simulink model "q3_model"  (R2020a)
settings: Solver=VariableStepAuto  StartTime=0.0  StopTime=10.0  RelTol=1e-3
libraries: simulink x1
settings Model: Creator=kiran  LastModifiedBy=kiran

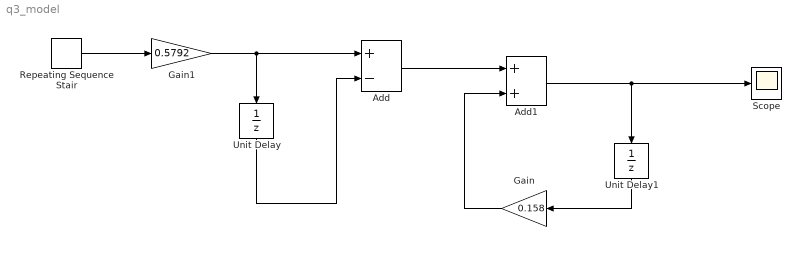
== system q3_model ==
  Add : Sum  Inputs=+-
  Add1 : Sum
  Gain : Gain  Gain=0.158
  Gain1 : Gain  Gain=0.5792
  Repeating Sequence Stair : simulink/Sources/Repeating Sequence Stair  OutValues=[1 0 0 0].'  tsamp=-1  OutMin=[]  OutMax=[]  OutDataTypeStr=double  OutputDataTypeScalingMode=double  OutDataType=fixdt(0,8)  ConRadixGroup=Best Precision: Vector-wise  OutScaling=2^-12
  Scope : Scope
  Unit Delay : UnitDelay  SampleTime=-1  HasFrameUpgradeWarning=on
  Unit Delay1 : UnitDelay  SampleTime=-1  HasFrameUpgradeWarning=on
  wires:
  Add1/1 -> Scope/1, Unit Delay1/1
  Add/1 -> Add1/1
  Unit Delay1/1 -> Gain/1
  Gain/1 -> Add1/2
  Repeating Sequence Stair/1 -> Gain1/1
  Gain1/1 -> Unit Delay/1, Add/1
  Unit Delay/1 -> Add/2
